simulink model "real_time_ecg"  (R2025a)
settings: Solver=FixedStepDiscrete  StartTime=0.0  StopTime=4.3200  FixedStep=0.008  RelTol=1e-3
undefined symbols (not defined in the file): ECG_max_amp
settings Model: Creator=DEV SONI  LastModifiedBy=DEV SONI

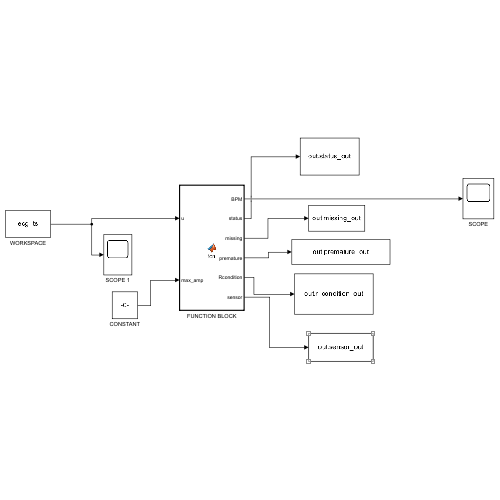
[thumbnail: Simulink's stored preview of the top-level diagram]
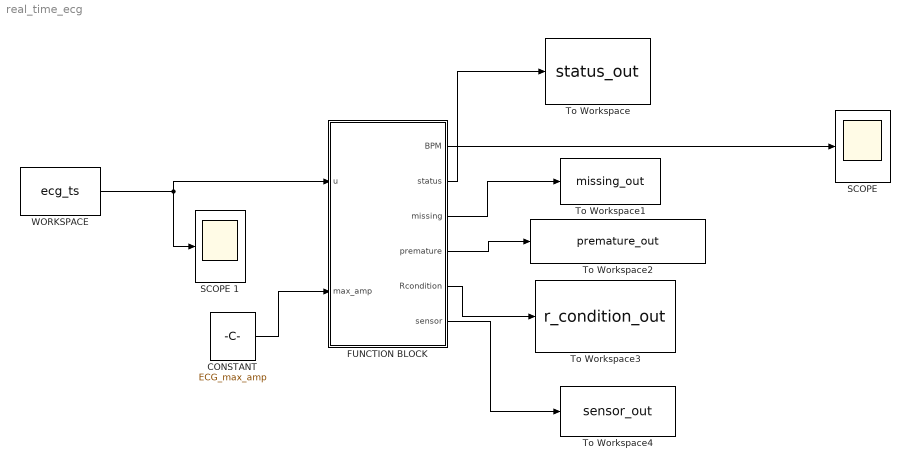
== system real_time_ecg ==
  CONSTANT : Constant  Value=ECG_max_amp
  FUNCTION BLOCK : MATLAB Function  TreatAsAtomicUnit=on
  SCOPE : Scope
      settings: ActiveDisplayYMinimum=-97.257681220221684  ActiveDisplayYMaximum=234.52849245662657
  SCOPE 1 : Scope
      settings: ActiveDisplayYMinimum=-0.212457379805653  ActiveDisplayYMaximum=1.1342196665601076
  To Workspace : ToWorkspace  VariableName=status_out  SampleTime=-1
  To Workspace1 : ToWorkspace  VariableName=missing_out  SampleTime=-1
  To Workspace2 : ToWorkspace  VariableName=premature_out  SampleTime=-1
  To Workspace3 : ToWorkspace  VariableName=r_condition_out  SampleTime=-1
  To Workspace4 : ToWorkspace  VariableName=sensor_out  SampleTime=-1
  WORKSPACE : FromWorkspace  VariableName=ecg_ts  SampleTime=1/125  OutputAfterFinalValue=Setting to zero
  wires:
  WORKSPACE/1 -> FUNCTION BLOCK/1(u), SCOPE 1/1
  FUNCTION BLOCK/1(BPM) -> SCOPE/1
  FUNCTION BLOCK/2(status) -> To Workspace/1
  FUNCTION BLOCK/3(missing) -> To Workspace1/1
  FUNCTION BLOCK/4(premature) -> To Workspace2/1
  FUNCTION BLOCK/5(Rcondition) -> To Workspace3/1
  FUNCTION BLOCK/6(sensor) -> To Workspace4/1
  CONSTANT/1 -> FUNCTION BLOCK/2(max_amp)

== matlab function real_time_ecg/FUNCTION BLOCK ==
  data: u input; BPM output; status output; missing output; premature output; Rcondition output; sensor output; max_amp input
function [BPM, status, missing, premature, Rcondition, sensor] = fcn(u, max_amp)

persistent prev last_peak sample ...
           early_count no_signal ...
           RR_hist peak_amp_hist ...
           missing_flag premature_flag ...
           real_beat_count ...
           status_flag Rcond_flag ...
           in_peak_region peak_max

if isempty(prev)
    prev            = 0;
    last_peak       = -1000;
    sample          = 0;
    early_count     = 0;
    no_signal       = 0;
    missing_flag    = 0;
    premature_flag  = 0;
    real_beat_count = 0;
    status_flag     = "Normal";
    Rcond_flag      = "Normal R Spike";
    in_peak_region  = 0;
    peak_max        = 0;
    RR_hist         = zeros(1, 8);
    peak_amp_hist   = zeros(1, 8);
end

sample = sample + 1;

BPM        = 0;
status     = status_flag;
missing    = "No Missing Beat";
premature  = "No Premature Beat";
Rcondition = Rcond_flag;
sensor     = "Sensor Connected";

% SENSOR DISCONNECT
if sample > 50
    if abs(u) < 0.01
        no_signal = no_signal + 1;
    else
        no_signal = 0;
    end
    if no_signal > 300
        sensor = "Sensor Disconnected";
        prev = u;
        return;
    end
end

% ADAPTIVE THRESHOLD
adaptive_thresh = 0.6 * max_amp;
min_refractory  = 25;

% PEAK AMPLITUDE TRACKING
if u > adaptive_thresh
    in_peak_region = 1;
    if u > peak_max
        peak_max = u;
    end
elseif in_peak_region == 1
    in_peak_region = 0;
    completed_peak_amp = peak_max;
    peak_max = 0;
    peak_amp_hist = [peak_amp_hist(2:end), completed_peak_amp];
    validPks = peak_amp_hist(peak_amp_hist > 0);
    if length(validPks) >= 3
        prev_mean = mean(validPks(1:end-1));
        curr_pk   = validPks(end);
        if curr_pk > 1.5 * prev_mean
            Rcond_flag = "High R Spike";
        elseif curr_pk < 0.5 * prev_mean
            Rcond_flag = "Weak R Spike";
        else
            Rcond_flag = "Normal R Spike";
        end
    end
end

% PEAK DETECTION
rising_edge     = (u > adaptive_thresh) && (prev <= adaptive_thresh);
past_refractory = ((sample - last_peak) > min_refractory);

if rising_edge && past_refractory
    if last_peak > 0

        RR_samples = sample - last_peak;

        % Compute mean from previous history BEFORE adding current
        validRR_prev = RR_hist(RR_hist > 0);
        if isempty(validRR_prev)
            meanRR_samples = RR_samples;
        else
            meanRR_samples = mean(validRR_prev);
        end

        % Update history
        RR_hist = [RR_hist(2:end), RR_samples];
        validRR = RR_hist(RR_hist > 0);

        % BPM — matches script: 60/mean(RR)
        BPM_now = 60 / (mean(validRR) / 125);

        % HEART RATE STATUS
        if BPM_now > 100
            status_flag = "Tachycardia";
        elseif BPM_now < 55
            status_flag = "Bradycardia";
        else
            status_flag = "Normal";
        end

        % Count real beats
        real_beat_count = real_beat_count + 1;

        % Only detect anomalies after 3 real beats
        if real_beat_count >= 2

            % MISSING BEAT
            if RR_samples > 1.5 * meanRR_samples
                missing_flag = 1;
            end

            % PREMATURE BEAT
            if RR_samples < 0.8 * meanRR_samples
                premature_flag = 1;
                early_count    = early_count + 1;
            else
                early_count = 0;
            end

            % REPEATED PREMATURE
            if early_count >= 2
                status_flag = "Repeated Premature Beats";
            end
        end
    end

    last_peak = sample;
end

% FINAL OUTPUTS
validRR_out = RR_hist(RR_hist > 0);
if ~isempty(validRR_out)
    BPM = 60 / (mean(validRR_out) / 125);
else
    BPM = 0;
end

status     = status_flag;
Rcondition = Rcond_flag;

if missing_flag == 1
    missing = "Missing Beat Detected";
end
if premature_flag == 1
    premature = "Premature Beat Detected";
end

prev = u;
end
